simulink model "s5_sim"  (R2022b)
settings: Solver=ode4  StartTime=0.0  StopTime=7  RelTol=1e-3
settings Model: Creator=kenobi  LastModifiedBy=kenobi
settings DataIOCC: ReturnWorkspaceOutputs=off

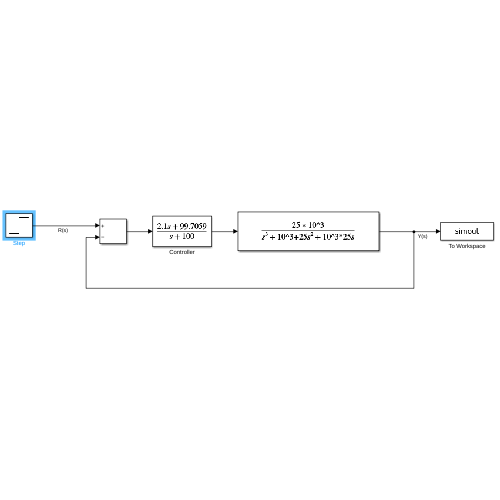
[thumbnail: Simulink's stored preview of the top-level diagram]
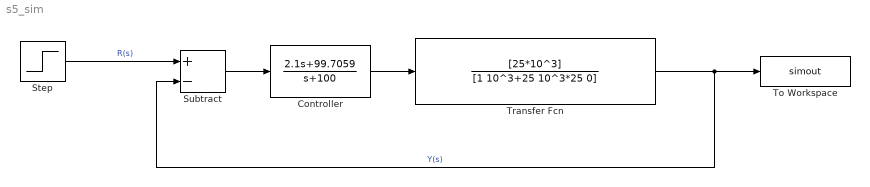
== system s5_sim ==
  Controller : TransferFcn  Numerator=[2.1 99.7059]  Denominator=[1 100]
  Step : Step  SampleTime=0
  Subtract : Sum  Inputs=+-
  To Workspace : ToWorkspace  VariableName=simout
      settings: Save2DSignal=2-D array (concatenate along first dimension)
  Transfer Fcn : TransferFcn  Numerator=[25*10^3]  Denominator=[1 10^3+25 10^3*25 0]
  wires:
  Controller/1 -> Transfer Fcn/1
  Transfer Fcn/1 -> Subtract/2, To Workspace/1  "Y(s)"
  Subtract/1 -> Controller/1
  Step/1 -> Subtract/1  "R(s)"
